simulink model "Verification_Tank2_Primitive"  (R2012b)
settings: Solver=FixedStepDiscrete  StartTime=0.0  StopTime=10.0  FixedStep=0.1  RelTol=1e-3
undefined symbols (not defined in the file): tank1_valve_flow_rate_m3s, tank2_cross_section_area_m2, tank2_e_valve_flow_rate_m3s, tank2_max_vol_m3, tank2_p_valve_flow_rate_m3s
libraries: sldvlib x19
settings Model: Creator=Kerianne  LastModifiedBy=Kerianne
settings DataIOCC: SaveFormat=Structure
settings OptimizationCC: InlineParams=on

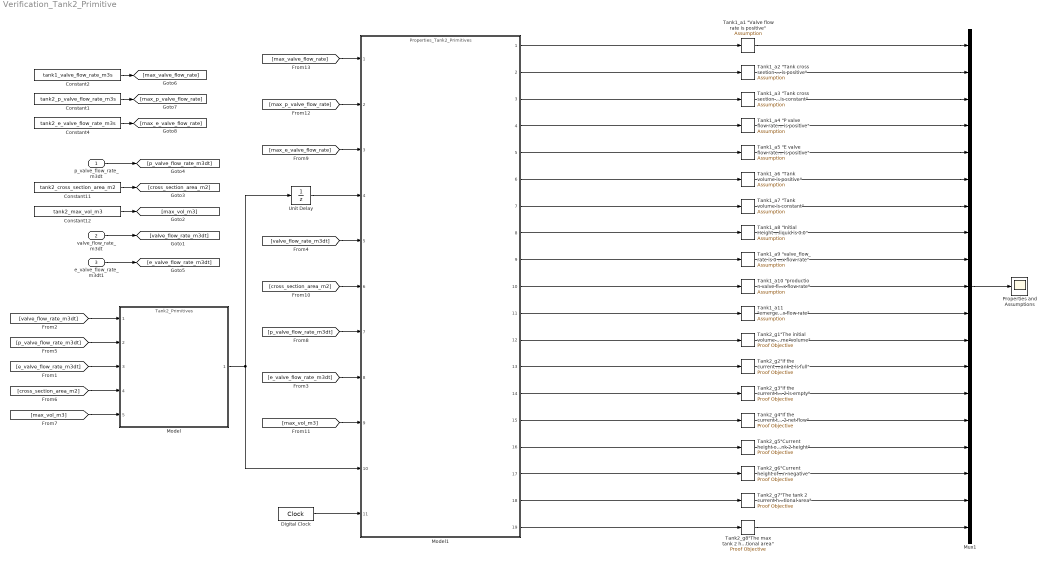
== system Verification_Tank2_Primitive ==
  p_valve_flow_rate_m3dt : Inport  OutDataTypeStr=double
  valve_flow_rate_m3dt : Inport  Port=2  OutDataTypeStr=double
  e_valve_flow_rate_m3dt1 : Inport  Port=3  OutDataTypeStr=double
  Constant1 : Constant  Value=tank2_p_valve_flow_rate_m3s
  Constant11 : Constant  Value=tank2_cross_section_area_m2
  Constant12 : Constant  Value=tank2_max_vol_m3
  Constant2 : Constant  Value=tank1_valve_flow_rate_m3s
  Constant4 : Constant  Value=tank2_e_valve_flow_rate_m3s
  Digital Clock : DigitalClock  SampleTime=0.1
  Model : ModelReference  ModelNameDialog=Tank2_Primitives  SimulationMode=Normal  ModelReferenceVersion=1.32  CopyOfModelName=Tank2_Primitives  DefaultDataLogging=on
  Model1 : ModelReference  ModelNameDialog=Properties_Tank2_Primitives  SimulationMode=Normal  ModelReferenceVersion=1.31  CopyOfModelName=Properties_Tank2_Primitives  DefaultDataLogging=on
  Mux1 : Mux  Inputs=19
  Properties and Assumptions : Scope
      settings: ShowLegends=on
  "Tank1_a1 \"Valve flow rate is positive\"" : sldvlib/Objectives and Constraints/Assumption  enabled=on  customAVTBlockType=Assumption  intervals=true  initial=off  dispValues=on  outEnabled=on
      settings: AttributesFormatString=%<intervals>
  "Tank1_a10 \"production valve flow rate is 0 or max flow rate\"" : sldvlib/Objectives and Constraints/Assumption  enabled=on  customAVTBlockType=Assumption  intervals=true  initial=off  dispValues=on  outEnabled=on
      settings: AttributesFormatString=%<intervals>
  "Tank1_a11 \"emergency valve flow rate is 0 or max flow rate\"" : sldvlib/Objectives and Constraints/Assumption  enabled=on  customAVTBlockType=Assumption  intervals=true  initial=off  dispValues=on  outEnabled=on
      settings: AttributesFormatString=%<intervals>
  "Tank1_a2 \"Tank cross section area is positive\"" : sldvlib/Objectives and Constraints/Assumption  enabled=on  customAVTBlockType=Assumption  intervals=true  initial=off  dispValues=on  outEnabled=on
      settings: AttributesFormatString=%<intervals>
  "Tank1_a3 \"Tank cross section area is constant\"" : sldvlib/Objectives and Constraints/Assumption  enabled=on  customAVTBlockType=Assumption  intervals=true  initial=off  dispValues=on  outEnabled=on
      settings: AttributesFormatString=%<intervals>
  "Tank1_a4 \"P valve flow rate is positive\"" : sldvlib/Objectives and Constraints/Assumption  enabled=on  customAVTBlockType=Assumption  intervals=true  initial=off  dispValues=on  outEnabled=on
      settings: AttributesFormatString=%<intervals>
  "Tank1_a5 \"E valve flow rate is positive\"" : sldvlib/Objectives and Constraints/Assumption  enabled=on  customAVTBlockType=Assumption  intervals=true  initial=off  dispValues=on  outEnabled=on
      settings: AttributesFormatString=%<intervals>
  "Tank1_a6 \"Tank volume is positive\"" : sldvlib/Objectives and Constraints/Assumption  enabled=on  customAVTBlockType=Assumption  intervals=true  initial=off  dispValues=on  outEnabled=on
      settings: AttributesFormatString=%<intervals>
  "Tank1_a7 \"Tank volume is constant\"" : sldvlib/Objectives and Constraints/Assumption  enabled=on  customAVTBlockType=Assumption  intervals=true  initial=off  dispValues=on  outEnabled=on
      settings: AttributesFormatString=%<intervals>
  "Tank1_a8 \"Initial Height of the liquid is 0.0\"" : sldvlib/Objectives and Constraints/Assumption  enabled=on  customAVTBlockType=Assumption  intervals=true  initial=off  dispValues=on  outEnabled=on
      settings: AttributesFormatString=%<intervals>
  "Tank1_a9 \"valve_flow_rate is 0 or max flow rate\"" : sldvlib/Objectives and Constraints/Assumption  enabled=on  customAVTBlockType=Assumption  intervals=true  initial=off  dispValues=on  outEnabled=on
      settings: AttributesFormatString=%<intervals>
  "Tank2_g1\"The initial volume of tank 2 should be equivalent to the specified initial tank 2 volume\"volume\" " : sldvlib/Objectives and Constraints/Proof Objective  enabled=on  customAVTBlockType=Proof Objective  intervals=true  dispValues=on  outEnabled=on  enableStopSim=off
      settings: AttributesFormatString=%<intervals>
  "Tank2_g2\"If the current tank 2 volume plus the tank 2 net flow is greater than the tank 2 maximum volume then tank 2 is full\"" : sldvlib/Objectives and Constraints/Proof Objective  enabled=on  customAVTBlockType=Proof Objective  intervals=true  dispValues=on  outEnabled=on  enableStopSim=off
      settings: AttributesFormatString=%<intervals>
  "Tank2_g3\"If the current tank 2 volume plus the tank 2 net flow is less than the tank 2 minimum volume then tank 2 is empty\"" : sldvlib/Objectives and Constraints/Proof Objective  enabled=on  customAVTBlockType=Proof Objective  intervals=true  dispValues=on  outEnabled=on  enableStopSim=off
      settings: AttributesFormatString=%<intervals>
  "Tank2_g4\"If the current tank 2 volume plus the tank 2 net flow is greater than empty and less than the tank 2 maximum volume then the tank 2 volume changes by the tank 2 net flow\"" : sldvlib/Objectives and Constraints/Proof Objective  enabled=on  customAVTBlockType=Proof Objective  intervals=true  dispValues=on  outEnabled=on  enableStopSim=off
      settings: AttributesFormatString=%<intervals>
  "Tank2_g5\"Current height of tank 2 is equal or less than the max tank 2 height\"" : sldvlib/Objectives and Constraints/Proof Objective  enabled=on  customAVTBlockType=Proof Objective  intervals=true  dispValues=on  outEnabled=on  enableStopSim=off
      settings: AttributesFormatString=%<intervals>
  "Tank2_g6\"Current height of tank 2 is non negative\"" : sldvlib/Objectives and Constraints/Proof Objective  enabled=on  customAVTBlockType=Proof Objective  intervals=true  dispValues=on  outEnabled=on  enableStopSim=off
      settings: AttributesFormatString=%<intervals>
  "Tank2_g7\"The tank 2 current height is equal to the tank 2 current volume divided by the tank 2 cross sectional area\" " : sldvlib/Objectives and Constraints/Proof Objective  enabled=on  customAVTBlockType=Proof Objective  intervals=true  dispValues=on  outEnabled=on  enableStopSim=off
      settings: AttributesFormatString=%<intervals>
  "Tank2_g8\"The max tank 2 height is equal to the max tank 2 volume divided by tank 2 cross sectional area\"" : sldvlib/Objectives and Constraints/Proof Objective  enabled=on  customAVTBlockType=Proof Objective  intervals=true  dispValues=on  outEnabled=on  enableStopSim=off
      settings: AttributesFormatString=%<intervals>
  Unit Delay : UnitDelay  SampleTime=-1
  wires:
  Model/1 -> Model1/10, Unit Delay/1
  Mux1/1 -> Properties and Assumptions/1
  valve_flow_rate_m3dt/1 -> [valve_flow_rate_m3dt]
  p_valve_flow_rate_m3dt/1 -> [p_valve_flow_rate_m3dt]
  Digital Clock/1 -> Model1/11
  e_valve_flow_rate_m3dt1/1 -> [e_valve_flow_rate_m3dt]
  [valve_flow_rate_m3dt] -> Model/1
  [p_valve_flow_rate_m3dt] -> Model/2
  [e_valve_flow_rate_m3dt] -> Model/3
  [cross_section_area_m2] -> Model/4
  [max_vol_m3] -> Model/5
  [valve_flow_rate_m3dt] -> Model1/5
  [cross_section_area_m2] -> Model1/6
  [p_valve_flow_rate_m3dt] -> Model1/7
  [e_valve_flow_rate_m3dt] -> Model1/8
  [max_vol_m3] -> Model1/9
  Model1/7 -> "Tank1_a7 \"Tank volume is constant\""/1
  Model1/6 -> "Tank1_a6 \"Tank volume is positive\""/1
  Model1/5 -> "Tank1_a5 \"E valve flow rate is positive\""/1
  Model1/4 -> "Tank1_a4 \"P valve flow rate is positive\""/1
  Model1/3 -> "Tank1_a3 \"Tank cross section area is constant\""/1
  Model1/2 -> "Tank1_a2 \"Tank cross section area is positive\""/1
  Model1/1 -> "Tank1_a1 \"Valve flow rate is positive\""/1
  "Tank1_a1 \"Valve flow rate is positive\""/1 -> Mux1/1
  "Tank1_a2 \"Tank cross section area is positive\""/1 -> Mux1/2
  "Tank1_a3 \"Tank cross section area is constant\""/1 -> Mux1/3
  "Tank1_a4 \"P valve flow rate is positive\""/1 -> Mux1/4
  "Tank1_a5 \"E valve flow rate is positive\""/1 -> Mux1/5
  "Tank1_a6 \"Tank volume is positive\""/1 -> Mux1/6
  "Tank1_a7 \"Tank volume is constant\""/1 -> Mux1/7
  Unit Delay/1 -> Model1/4
  Constant11/1 -> [cross_section_area_m2]
  Constant12/1 -> [max_vol_m3]
  Constant2/1 -> [max_valve_flow_rate]
  Constant1/1 -> [max_p_valve_flow_rate]
  Constant4/1 -> [max_e_valve_flow_rate]
  [max_e_valve_flow_rate] -> Model1/3
  [max_p_valve_flow_rate] -> Model1/2
  [max_valve_flow_rate] -> Model1/1
  Model1/11 -> "Tank1_a11 \"emergency valve flow rate is 0 or max flow rate\""/1
  Model1/10 -> "Tank1_a10 \"production valve flow rate is 0 or max flow rate\""/1
  Model1/9 -> "Tank1_a9 \"valve_flow_rate is 0 or max flow rate\""/1
  Model1/8 -> "Tank1_a8 \"Initial Height of the liquid is 0.0\""/1
  "Tank1_a8 \"Initial Height of the liquid is 0.0\""/1 -> Mux1/8
  "Tank1_a9 \"valve_flow_rate is 0 or max flow rate\""/1 -> Mux1/9
  "Tank1_a10 \"production valve flow rate is 0 or max flow rate\""/1 -> Mux1/10
  "Tank1_a11 \"emergency valve flow rate is 0 or max flow rate\""/1 -> Mux1/11
  Model1/12 -> "Tank2_g1\"The initial volume of tank 2 should be equivalent to the specified initial tank 2 volume\"volume\" "/1
  "Tank2_g1\"The initial volume of tank 2 should be equivalent to the specified initial tank 2 volume\"volume\" "/1 -> Mux1/12
  Model1/13 -> "Tank2_g2\"If the current tank 2 volume plus the tank 2 net flow is greater than the tank 2 maximum volume then tank 2 is full\""/1
  "Tank2_g2\"If the current tank 2 volume plus the tank 2 net flow is greater than the tank 2 maximum volume then tank 2 is full\""/1 -> Mux1/13
  Model1/14 -> "Tank2_g3\"If the current tank 2 volume plus the tank 2 net flow is less than the tank 2 minimum volume then tank 2 is empty\""/1
  "Tank2_g3\"If the current tank 2 volume plus the tank 2 net flow is less than the tank 2 minimum volume then tank 2 is empty\""/1 -> Mux1/14
  Model1/15 -> "Tank2_g4\"If the current tank 2 volume plus the tank 2 net flow is greater than empty and less than the tank 2 maximum volume then the tank 2 volume changes by the tank 2 net flow\""/1
  "Tank2_g4\"If the current tank 2 volume plus the tank 2 net flow is greater than empty and less than the tank 2 maximum volume then the tank 2 volume changes by the tank 2 net flow\""/1 -> Mux1/15
  Model1/16 -> "Tank2_g5\"Current height of tank 2 is equal or less than the max tank 2 height\""/1
  "Tank2_g5\"Current height of tank 2 is equal or less than the max tank 2 height\""/1 -> Mux1/16
  Model1/17 -> "Tank2_g6\"Current height of tank 2 is non negative\""/1
  "Tank2_g6\"Current height of tank 2 is non negative\""/1 -> Mux1/17
  Model1/18 -> "Tank2_g7\"The tank 2 current height is equal to the tank 2 current volume divided by the tank 2 cross sectional area\" "/1
  "Tank2_g7\"The tank 2 current height is equal to the tank 2 current volume divided by the tank 2 cross sectional area\" "/1 -> Mux1/18
  Model1/19 -> "Tank2_g8\"The max tank 2 height is equal to the max tank 2 volume divided by tank 2 cross sectional area\""/1
  "Tank2_g8\"The max tank 2 height is equal to the max tank 2 volume divided by tank 2 cross sectional area\""/1 -> Mux1/19
